simulink model "tpireloaded"  (R2017b)
settings: Solver=FixedStepAuto  StartTime=0.0  StopTime=1  FixedStep=1e-6  MaxStep=1e-4  RelTol=1e-3
values from neighbouring files (symbols this model uses):
  dcin = 547.66    [tpi2parallelrunner.m]    (also in tpi2seriesrunner.m = 20; tpireloadedrunner.m)
  Ef = 154.55/2    (= 77.275)    [tpireloadedrunner.m]
  fdclinkres = 1e-6    (= 1e-06)    [tpi2parallelrunner.m]    (also in tpi2seriesrunner.m; tpireloadedrunner.m)
  fma = 0.9    [tpi2parallelrunner.m]    (also in tpi2seriesrunner.m; tpireloadedrunner.m)
  Rin = 1    [tpi2parallelrunner.m]    (also in tpi2seriesrunner.m = 1e-16; tpireloadedrunner.m)
  sdclinkcap = 1e-2    (= 0.01)    [tpi2seriesrunner.m]    (also in tpireloadedrunner.m)
  SLload = SXload/sreffreq    [tpi2parallelrunner.m]    (also in tpi2seriesrunner.m = 0.002; tpireloadedrunner.m)
  sma = 0.9    [tpi2parallelrunner.m]    (also in tpi2seriesrunner.m; tpireloadedrunner.m)
  sreffreq = 2*pi*50    (= 314.159265359)    [tpi2parallelrunner.m]    (also in tpi2seriesrunner.m; tpireloadedrunner.m)
  SRload = SZload*Load_Power_Factor    [tpi2parallelrunner.m]    (also in tpi2seriesrunner.m = 5; tpireloadedrunner.m = n*SZload*Load_Power_Factor)
undefined symbols (not defined in the file or in its folder): fdclink1cap
libraries: powerlib x28, dspstat3 x4, powerlib_meascontrol x3, simulink x3
settings Model: SimulationMode=rapid-accelerator  Creator=Orhun  LastModifiedBy=Orhun

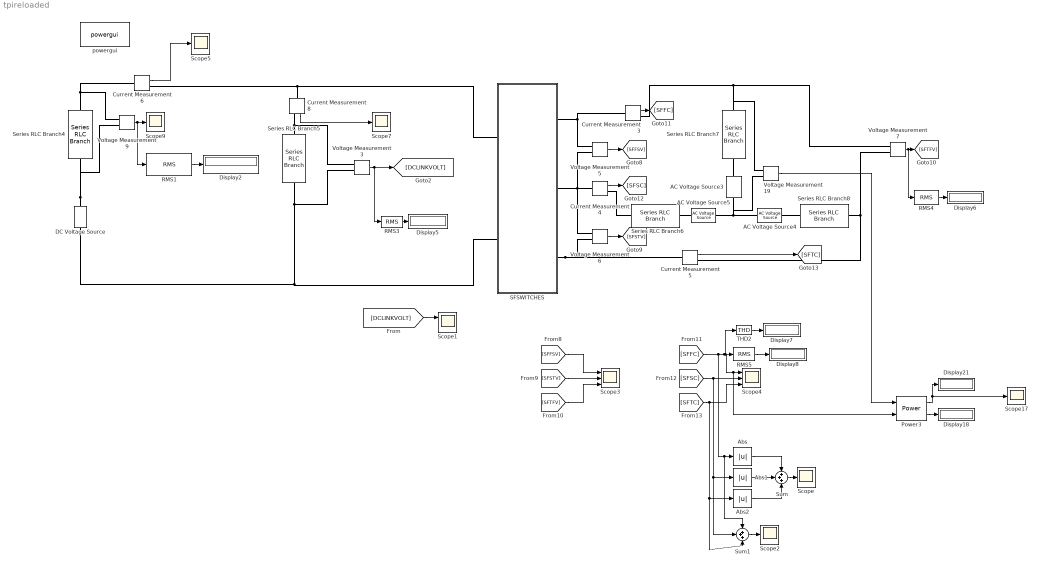
== system tpireloaded ==
  AC Voltage Source3 : powerlib/Electrical Sources/AC Voltage Source  Amplitude=Ef*sqrt(2)  Phase=0  Frequency=sreffreq  SampleTime=0  Measurements=None  BusType=swing  Pref=10e3  Qref=0  Qmin=-inf  Qmax=+inf
  AC Voltage Source4 : powerlib/Electrical Sources/AC Voltage Source  Amplitude=Ef*sqrt(2)  Phase=-2*pi/3  Frequency=sreffreq  SampleTime=0  Measurements=None  BusType=swing  Pref=10e3  Qref=0  Qmin=-inf  Qmax=+inf
  AC Voltage Source5 : powerlib/Electrical Sources/AC Voltage Source  Amplitude=Ef*sqrt(2)  Phase=2*pi/3  Frequency=sreffreq  SampleTime=0  Measurements=None  BusType=swing  Pref=10e3  Qref=0  Qmin=-inf  Qmax=+inf
  Abs : Abs
  Abs1 : Abs
  Abs2 : Abs
  Current Measurement{3..6,8} (5 alike) : powerlib/Measurements/Current Measurement  PhasorSimulation=off  OutputType=Complex  PSBequivalent=0
  DC Voltage Source : powerlib/Electrical Sources/DC Voltage Source  Amplitude=dcin  Measurements=None
  Display{2,5..8,18,21} (7 alike) : Display
  Power3 : powerlib_meascontrol/Measurements/Power  Freq=60  Vinit=[1, 0]  Iinit=[1, 0]  Ts=0
      settings: SourceProductName=Simscape Power Systems
  RMS1 : dspstat3/RMS  run=off  directionMode=Each column  dimension=1  InputProcessing=Columns as channels (frame based)  reset_popup=None
  RMS3 : dspstat3/RMS  run=off  directionMode=Each column  dimension=1  InputProcessing=Columns as channels (frame based)  reset_popup=None
  RMS4 : dspstat3/RMS  run=on  directionMode=Entire input  dimension=1  InputProcessing=Columns as channels (frame based)  reset_popup=None
  RMS5 : dspstat3/RMS  run=on  directionMode=Entire input  dimension=1  InputProcessing=Columns as channels (frame based)  reset_popup=None
  SFSWITCHES : Subsystem
  Scope{,2,5,7,9,17} (6 alike) : Scope
  Scope1 : Scope  NumInputPorts=2
  Scope3 : Scope  NumInputPorts=3
  Scope4 : Scope  NumInputPorts=3
  Series RLC Branch4 : powerlib/Elements/Series RLC Branch  LConnTagsString=__new0  RConnTagsString=__new0  BranchType=R  Resistance=Rin  Inductance=0  SetiL0=off  InitialCurrent=0  Capacitance=fdclink1cap  Setx0=off  InitialVoltage=0  Measurements=None
  Series RLC Branch5 : powerlib/Elements/Series RLC Branch  LConnTagsString=__new0  RConnTagsString=__new0  BranchType=C  Resistance=fdclinkres  Inductance=0  SetiL0=off  InitialCurrent=0  Capacitance=sdclinkcap  Setx0=off  InitialVoltage=dcin/2  Measurements=None
  Series RLC Branch6 : powerlib/Elements/Series RLC Branch  LConnTagsString=__new0  RConnTagsString=__new0  BranchType=RL  Resistance=SRload  Inductance=SLload  SetiL0=off  InitialCurrent=0  Capacitance=0  Setx0=off  InitialVoltage=0  Measurements=None
  Series RLC Branch7 : powerlib/Elements/Series RLC Branch  LConnTagsString=__new0  RConnTagsString=__new0  BranchType=RL  Resistance=SRload  Inductance=SLload  SetiL0=off  InitialCurrent=0  Capacitance=0  Setx0=off  InitialVoltage=0  Measurements=None
  Series RLC Branch8 : powerlib/Elements/Series RLC Branch  LConnTagsString=__new0  RConnTagsString=__new0  BranchType=RL  Resistance=SRload  Inductance=SLload  SetiL0=off  InitialCurrent=0  Capacitance=0  Setx0=off  InitialVoltage=0  Measurements=None
  Sum : Sum  Inputs=+++
  Sum1 : Sum  Inputs=+++
  THD2 : powerlib_meascontrol/Measurements/THD  Freq=50  Ts=0
  Voltage Measurement{3,5..7,9,19} (6 alike) : powerlib/Measurements/Voltage Measurement  PhasorSimulation=off  OutputType=Complex  PSBequivalent=0
  powergui : powerlib/powergui  Priority=1  SimulationMode=Discrete  SampleTime=1e-6  frequency=60  Iterations=50  frequencyindice=0  Pbase=100e6  ErrMax=1e-4  UnitsV=kV  UnitsW=MW  buscounter=0  FunctionMessages=on  echomessages=off  EnableUseOfTLC=off  CurrentSourceSwitches=off  DisableSnubberDevices=off  DisableRonSwitches=off  DisableVfSwitches=off  DisplayEquations=off  SolverType=Tustin/Backward Euler (TBE)  Interpol=off  ExternalGateDelay=off  methode=off  Ts=100  x0status=blocks  SPID=off  SwTol=0  HookPort=off  RestoreLinks=warning  ResistiveCurrentMeasurement=off  Frange=[0:2:500]  Ylog=off  Xlog=on  ShowGrid=off  save=off  variable=ZData  structure=0  ZoomFFT=off  StartTime=0.0  cycles=1  DisplayStyle=1  fundamental=60  FreqAxis=off  MaxFrequency=1000  frequencyindicesteady=1  RmsSteady=1  display=off
  wires:
  Voltage Measurement19/1 -> Power3/1
  RMS5/1 -> Display8/1
  Current Measurement4/1 -> [SFSC]
  Voltage Measurement3/1 -> RMS3/1, [DCLINKVOLT]
  Voltage Measurement5/1 -> [SFFSV]
  Voltage Measurement7/1 -> RMS4/1, [SFTFV]
  Current Measurement8/1 -> Scope7/1
  RMS3/1 -> Display5/1
  [SFTFV] -> Scope3/3
  [SFSTV] -> Scope3/2
  [SFFSV] -> Scope3/1
  Current Measurement5/1 -> [SFTC]
  Current Measurement3/1 -> [SFFC]
  Voltage Measurement6/1 -> [SFSTV]
  THD2/1 -> Display7/1
  Power3/1 -> Display21/1, Scope17/1
  RMS4/1 -> Display6/1
  Power3/2 -> Display18/1
  [DCLINKVOLT] -> Scope1/1
  RMS1/1 -> Display2/1
  Voltage Measurement9/1 -> RMS1/1, Scope9/1
  Current Measurement6/1 -> Scope5/1
  [SFSC] -> Sum1/2, Abs1/1, Scope4/2
  Abs/1 -> Sum/1
  [SFTC] -> Sum1/3, Abs2/1, Scope4/3
  Abs2/1 -> Sum/3
  Sum/1 -> Scope/1
  [SFFC] -> Sum1/1, Abs/1, Power3/2, Scope4/1, THD2/1, RMS5/1
  Abs1/1 -> Sum/2
  Sum1/1 -> Scope2/1
  connections:
  SFSWITCHES/RConn3 -- Voltage Measurement6/LConn2 -- Current Measurement5/LConn1
  Current Measurement5/RConn1 -- Series RLC Branch8/LConn1 -- Voltage Measurement7/LConn1
  AC Voltage Source5/LConn1 -- AC Voltage Source4/LConn1 -- AC Voltage Source3/LConn1 -- Voltage Measurement19/LConn2
  Series RLC Branch5/LConn1 -- Current Measurement8/RConn1 -- Voltage Measurement3/LConn1
  Series RLC Branch5/RConn1 -- Voltage Measurement3/LConn2 -- DC Voltage Source/LConn1 -- SFSWITCHES/LConn2
  Voltage Measurement7/LConn2 -- Current Measurement3/RConn1 -- Voltage Measurement19/LConn1 -- Series RLC Branch7/RConn1
  Current Measurement3/LConn1 -- Voltage Measurement5/LConn1 -- SFSWITCHES/RConn1
  Voltage Measurement6/LConn1 -- Voltage Measurement5/LConn2 -- SFSWITCHES/RConn2 -- Current Measurement4/LConn1
  AC Voltage Source5/RConn1 -- Series RLC Branch6/LConn1
  Series RLC Branch6/RConn1 -- Current Measurement4/RConn1
  AC Voltage Source3/RConn1 -- Series RLC Branch7/LConn1
  AC Voltage Source4/RConn1 -- Series RLC Branch8/RConn1
  Current Measurement8/LConn1 -- SFSWITCHES/LConn1 -- Current Measurement6/RConn1
  DC Voltage Source/RConn1 -- Series RLC Branch4/RConn1 -- Voltage Measurement9/LConn2
  Current Measurement6/LConn1 -- Voltage Measurement9/LConn1 -- Series RLC Branch4/LConn1

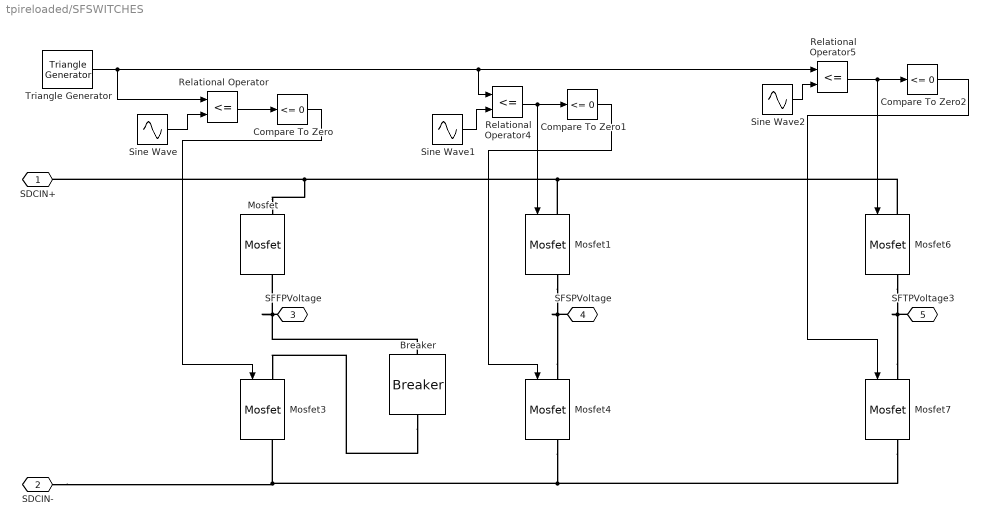
== system tpireloaded/SFSWITCHES ==
  Breaker : powerlib/Elements/Breaker  InitialState=1  SwitchingTimes=0.055  External=off  BreakerResistance=1e-6  SnubberResistance=1e6  SnubberCapacitance=inf  Measurements=None  MoreParameters=on  NoBreakLoop=off
      settings: SourceProductName=Simscape Power Systems
  Compare To Zero : simulink/Logic and Bit Operations/Compare To Zero  relop=<=  OutDataTypeStr=boolean
  Compare To Zero1 : simulink/Logic and Bit Operations/Compare To Zero  relop=<=  OutDataTypeStr=boolean
  Compare To Zero2 : simulink/Logic and Bit Operations/Compare To Zero  relop=<=  OutDataTypeStr=boolean
  Mosfet{,1,3..4,6..7} (6 alike) : powerlib/Power Electronics/Mosfet  Ron=2e-3  Lon=0  Rd=0.01  Vfd=0  IC=0  Rs=1e5  Cs=inf  Measurements=on
  Relational Operator : RelationalOperator  Operator=<=  OutDataTypeStr=boolean  RndMeth=Simplest
  Relational Operator4 : RelationalOperator  Operator=<=  OutDataTypeStr=boolean  RndMeth=Simplest
  Relational Operator5 : RelationalOperator  Operator=<=  OutDataTypeStr=boolean  RndMeth=Simplest
  Sine Wave : Sin  Amplitude=sma  Frequency=sreffreq  SampleTime=0
  Sine Wave1 : Sin  Amplitude=sma  Frequency=sreffreq  Phase=2*pi/3  SampleTime=0
  Sine Wave2 : Sin  Amplitude=fma  Frequency=sreffreq  Phase=4*pi/3  SampleTime=0
  Triangle Generator : powerlib_meascontrol/Pulse & Signal Generators/Triangle Generator  Freq=sswfreq  Phase=270  Ts=1e-6
  SDCIN+ : PMIOPort  Port=1  Side=Left
  SDCIN- : PMIOPort  Port=2  Side=Left
  SFFPVoltage : PMIOPort  Port=3  Side=Right
  SFSPVoltage : PMIOPort  Port=4  Side=Right
  SFTPVoltage3 : PMIOPort  Port=5  Side=Right
  wires:
  Sine Wave/1 -> Relational Operator/2
  Triangle Generator/1 -> Relational Operator5/1, Relational Operator4/1, Relational Operator/1
  Relational Operator4/1 -> Mosfet1/1, Compare To Zero1/1
  Sine Wave2/1 -> Relational Operator5/2
  Sine Wave1/1 -> Relational Operator4/2
  Relational Operator/1 -> Compare To Zero/1
  Compare To Zero/1 -> Mosfet3/1
  Compare To Zero1/1 -> Mosfet4/1
  Compare To Zero2/1 -> Mosfet7/1
  Relational Operator5/1 -> Mosfet6/1, Compare To Zero2/1
  connections:
  Mosfet7/LConn1 -- Mosfet6/RConn1 -- SFTPVoltage3/RConn1
  SFFPVoltage/RConn1 -- Breaker/LConn1 -- Mosfet/RConn1
  Mosfet4/LConn1 -- Mosfet1/RConn1 -- SFSPVoltage/RConn1
  Mosfet4/RConn1 -- Mosfet3/RConn1 -- SDCIN-/RConn1 -- Mosfet7/RConn1
  Mosfet/LConn1 -- SDCIN+/RConn1 -- Mosfet6/LConn1 -- Mosfet1/LConn1
  Breaker/RConn1 -- Mosfet3/LConn1
